simulink model "practica2"  (Simulink 6.2)
settings: Solver=ode45  StartTime=0.0  StopTime=10.0  RelTol=1e-3
undefined symbols (not defined in the file or in its folder): amp
settings Model: LastModifiedBy=rolimat  ExtModeTrigMode=oneshot  ExtModeArmWhenConnect=off
settings DataIOCC: LimitDataPoints=off
settings OptimizationCC: BlockReduction=off  BooleanDataType=off
settings HardwareCC: TargetUnknown=on
settings STFCustomTargetCC: TargetFcnLib=ansi_tfl_tmw.mat  GenFloatMathFcnCalls=ANSI_C  ModelReferenceCompliant=off  SystemTargetFile=grt.tlc

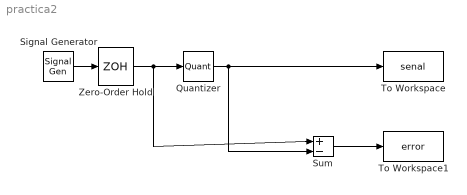
== system practica2 ==
  Quantizer : Quantizer  QuantizationInterval=2*10/2^5
  Signal Generator : SignalGenerator  Amplitude=amp  Frequency=10
  Sum : Sum  Inputs=|+-  SaturateOnIntegerOverflow=on  InputSameDT=on
  To Workspace : ToWorkspace  VariableName=senal  SampleTime=-1  SaveFormat=Array
  To Workspace1 : ToWorkspace  VariableName=error  SampleTime=-1  SaveFormat=Array
  Zero-Order Hold : ZeroOrderHold  SampleTime=0.01
  wires:
  Sum/1 -> To Workspace1/1
  Quantizer/1 -> Sum/2, To Workspace/1
  Signal Generator/1 -> Zero-Order Hold/1
  Zero-Order Hold/1 -> Quantizer/1, Sum/1
